simulink model "CAN_Model_FrameFormatter"  (R2018b)
settings: Solver=VariableStepAuto  StartTime=0.0  StopTime=1.0  RelTol=1e-3
InitFcn:
  | clc;
  | clear;
settings Model: Creator=Emiliano  LastModifiedBy=MAX_1
settings DebuggingCC: LibraryContextMissingDiagnostic=none
settings SFSimCC: SimUseLocalCustomCode=off
settings RTWCC: RTWUseLocalCustomCode=off

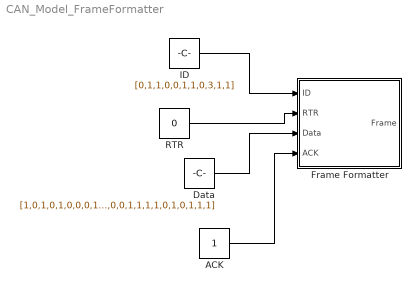
== system CAN_Model_FrameFormatter ==
  ACK : Constant
  "Data " : Constant  Value=[1,0,1,0,1,0,0,0,1,1,0,1,0,1,0,1,0,1,0,1,0,1,0,1,0,1,0,1,1,1,1,1,1,1,1,1,1,1,1,1,1,1,1,1,1,0,0,0,0,0,0,0,0,0,1,1,1,1,0,1,0,1,1,1]
  Frame Formatter : Subsystem
  ID : Constant  Value=[0,1,1,0,0,1,1,0,3,1,1]  SampleTime=0.000002
  RTR : Constant  Value=0
  wires:
  ID/1 -> Frame Formatter/1(ID)
  RTR/1 -> Frame Formatter/2(RTR)
  "Data "/1 -> Frame Formatter/3(Data)
  ACK/1 -> Frame Formatter/4(ACK)

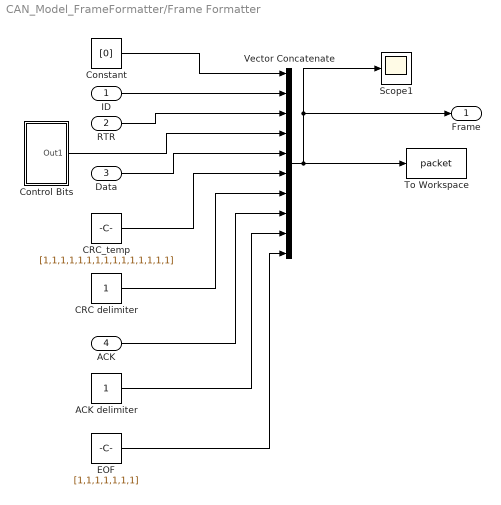
== system CAN_Model_FrameFormatter/Frame Formatter ==
  ID : Inport
  RTR : Inport  Port=2
  Data : Inport  Port=3
  ACK : Inport  Port=4
  ACK delimiter : Constant
  CRC delimiter : Constant  VectorParams1D=off
  CRC_temp : Constant  Value=[1,1,1,1,1,1,1,1,1,1,1,1,1,1,1]
  Constant : Constant  Value=[0]  SampleTime=0.000002
  Control Bits : Subsystem
  EOF : Constant  Value=[1,1,1,1,1,1,1]  SampleTime=0.000002
  Scope1 : Scope
  To Workspace : ToWorkspace  VariableName=packet  SaveFormat=Timeseries  SampleTime=-1
  Vector Concatenate : Concatenate  NumInputs=10
  Frame : Outport
  wires:
  ID/1 -> Vector Concatenate/2
  Constant/1 -> Vector Concatenate/1
  Data/1 -> Vector Concatenate/5
  Vector Concatenate/1 -> Scope1/1, Frame/1, To Workspace/1
  RTR/1 -> Vector Concatenate/3
  Control Bits/1(Out1) -> Vector Concatenate/4
  CRC_temp/1 -> Vector Concatenate/6
  CRC delimiter/1 -> Vector Concatenate/7
  ACK/1 -> Vector Concatenate/8
  ACK delimiter/1 -> Vector Concatenate/9
  EOF/1 -> Vector Concatenate/10

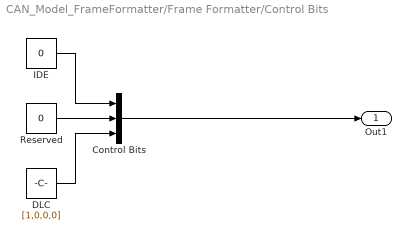
== system CAN_Model_FrameFormatter/Frame Formatter/Control Bits ==
  Control Bits : Concatenate  NumInputs=3
  DLC : Constant  Value=[1,0,0,0]
  IDE : Constant  Value=0
  Reserved : Constant  Value=0
  Out1 : Outport
  wires:
  DLC/1 -> Control Bits/3
  IDE/1 -> Control Bits/1
  Reserved/1 -> Control Bits/2
  Control Bits/1 -> Out1/1
